simulink model "z_dod_symulacja"  (R2021a)
settings: Solver=VariableStepAuto  StartTime=0.0  StopTime=35  RelTol=1e-3
values from neighbouring files (symbols this model uses):
  k1 = k(1)    [z_dod.m]
  k2 = k(2)    [z_dod.m]
  k3 = k(3)    [z_dod.m]
  k4 = k(4)    [z_dod.m]
settings Model: Creator=48604  LastModifiedBy=48604

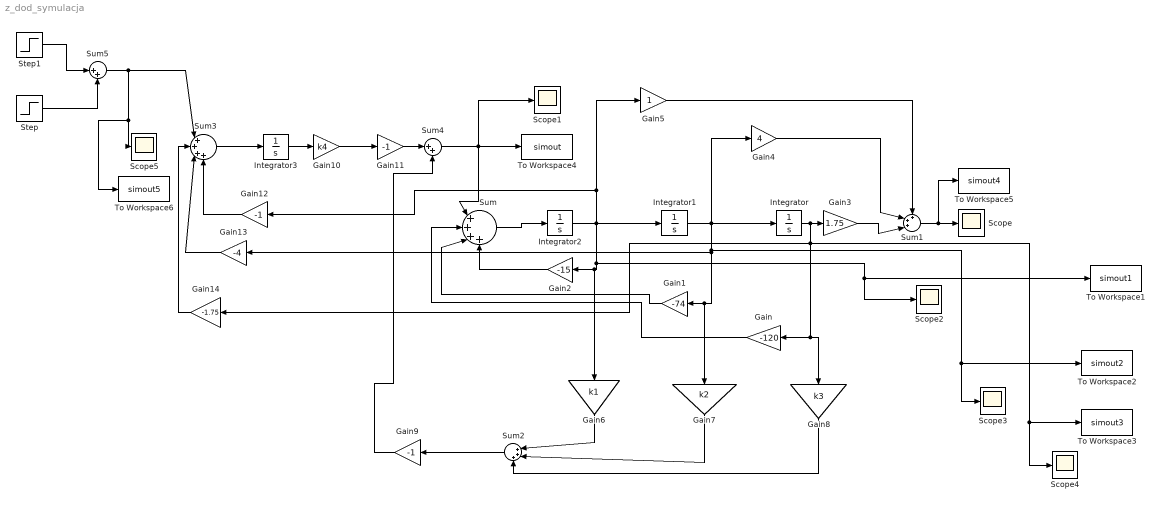
== system z_dod_symulacja ==
  Gain : Gain  Gain=-120
  Gain1 : Gain  Gain=-74
  Gain10 : Gain  Gain=k4
  Gain11 : Gain  Gain=-1
  Gain12 : Gain  Gain=-1
  Gain13 : Gain  Gain=-4
  Gain14 : Gain  Gain=-1.75
  Gain2 : Gain  Gain=-15
  Gain3 : Gain  Gain=1.75
  Gain4 : Gain  Gain=4
  Gain5 : Gain
  Gain6 : Gain  Gain=k1
  Gain7 : Gain  Gain=k2
  Gain8 : Gain  Gain=k3
  Gain9 : Gain  Gain=-1
  Integrator{,1..3} (4 alike) : Integrator
  Scope{,1..5} (6 alike) : Scope
  Step : Step  Time=2  After=4  SampleTime=0
  Step1 : Step  Time=8  After=-4  SampleTime=1
  Sum : Sum  Inputs=|++++
  Sum1 : Sum  Inputs=+++|
  Sum2 : Sum  Inputs=|+++
  Sum3 : Sum  Inputs=|++++
  Sum4 : Sum  Inputs=|++
  Sum5 : Sum  Inputs=|++
  To Workspace1 : ToWorkspace  VariableName=simout1  SaveFormat=Structure With Time  SampleTime=-1
  To Workspace2 : ToWorkspace  VariableName=simout2  SaveFormat=Structure With Time  SampleTime=-1
  To Workspace3 : ToWorkspace  VariableName=simout3  SaveFormat=Structure With Time  SampleTime=-1
  To Workspace4 : ToWorkspace  VariableName=simout  SaveFormat=Structure With Time  SampleTime=-1
  To Workspace5 : ToWorkspace  VariableName=simout4  SaveFormat=Structure With Time  SampleTime=-1
  To Workspace6 : ToWorkspace  VariableName=simout5  SaveFormat=Structure With Time  SampleTime=-1
  wires:
  Gain1/1 -> Sum/3
  Gain7/1 -> Sum2/2
  Sum1/1 -> To Workspace5/1, Scope/1
  Gain6/1 -> Sum2/1
  Integrator2/1 -> Gain12/1, Gain5/1, Scope2/1, To Workspace1/1, Gain2/1, Gain6/1, Integrator1/1
  Gain3/1 -> Sum1/3
  Integrator/1 -> Gain14/1, To Workspace3/1, Scope4/1, Gain8/1, Gain/1, Gain3/1
  Gain/1 -> Sum/2
  Integrator1/1 -> Gain13/1, Gain7/1, Gain1/1, To Workspace2/1, Scope3/1, Gain4/1, Integrator/1
  Gain5/1 -> Sum1/1
  Sum2/1 -> Gain9/1
  Sum/1 -> Integrator2/1
  Gain2/1 -> Sum/4
  Gain8/1 -> Sum2/3
  Gain4/1 -> Sum1/2
  Integrator3/1 -> Gain10/1
  Gain10/1 -> Gain11/1
  Sum3/1 -> Integrator3/1
  Gain12/1 -> Sum3/4
  Gain13/1 -> Sum3/3
  Gain14/1 -> Sum3/2
  Sum4/1 -> Scope1/1, To Workspace4/1, Sum/1
  Gain9/1 -> Sum4/2
  Gain11/1 -> Sum4/1
  Step1/1 -> Sum5/1
  Step/1 -> Sum5/2
  Sum5/1 -> To Workspace6/1, Scope5/1, Sum3/1
